simulink library "MIL_Test"  (Simulink 6.6)
undefined symbols (not defined in the file or in its folder): getdatatypespecs, slcm, StepSize
libraries: simulink x71, MIL_Test x6
(part 5 of 8)

== system MIL_Test/Validation Function/Feature extraction/Step response characteristics/Step response characteristics extraction/Extract maximum overshoot/Step response moving average and initial conditions before step ==
  Reset : Inport
  Step response : Inport  Port=2
  Add2 : Sum  Inputs=+-  OutScaling=2^-10
  Constant : Constant  Value=0
  Flip if new step : Subsystem  TreatAsAtomicUnit=on
  Memory : Memory
  Switch : Switch  Criteria=u2 ~= 0
  Switch1 : Switch  Criteria=u2 ~= 0
  Switch2 : Switch  Criteria=u2 ~= 0
  Weighted Moving Average : S-Function  FunctionName=sfix_fir  Parameters=(getdatatypespecs(OutDataType,OutScaling,DblOver,0)),[DoSatur RndMeth-1],DblOver,dolog,mgainval,(getdatatypespecs(GainDataType,GainScaling,DblOver,RadixGroup)),samptime,vinit,OutputDataTypeScalingMode,GainDataTypeScalingMode  mask(Weighted Moving Average){mgainval=ones(1,10), vinit=0.0, samptime=-1, GainDataTypeScalingMode=Inherit via internal rule, GainDataType=sfix( 16 ), MatRadixGroup=Best Precision: Matrix-wise, GainScaling=2^-10, OutputDataTypeScalingMode=Inherit via internal rule, OutDataType=sfix(16), OutScaling=2^-10, LockScale=off, RndMeth=Floor, DoSatur=off}
      mask prompts: mgainval "Weights:"; vinit "Initial condition:"; samptime "Sample time:"; GainDataTypeScalingMode "Gain data type and scaling:"; GainDataType "Parameter data type:     ex. sfix(16),  uint(8), float('single')"; MatRadixGroup "Parameter scaling mode:"; GainScaling "Parameter scaling:    Slope    ex.  2^-9"; OutputDataTypeScalingMode "Output data type and scaling:"; OutDataType "Output data type:     ex.  sfix(16),  uint(8),  float('single')"; OutScaling "Output scaling:    Slope or [Slope Bias]    ex.  2^-9"; LockScale "Lock output scaling so autoscaling tool can't change it"; RndMeth "Round toward:"; DoSatur "Saturate to max or min when overflows occur"
      mask help: Output the weighted moving average of the input.
      mask init: same as MIL_Test/Validation Function/Feature extraction/Step response characteristics/Step response characteristics extraction/Extract steady state error/Weighted Moving Average
      mask StyleString: edit,edit,edit,popup(Specify via dialog|Inherit via internal rule),edit,popup(Use Specified Scaling|Best Precision: Element-wise|Best Precision: Row-wise|Best Precision: Column-wise|Best Precision: Matrix-wise),edit,popup(Specify via dialog|Inherit via internal rule|Inherit via back propagation),edit,edit,checkbox,popup(Zero|Nearest|Ceiling|Floor),checkbox
      mask CallbackString: |||fixptdialog(gcbh)|fixptdialog(gcbh)|fixptdialog(gcbh)||fixptdialog(gcbh)|fixptdialog(gcbh)||||
      mask TabNameString: Main,Main,Main,Parameter data types,Parameter data types,Parameter data types,Parameter data types,Signal data types,Signal data types,Signal data types,Signal data types,Signal data types,Signal data types
      mask Display:
      | fprintf(fixpt_fir_mask_data(mgainval,'dispstr'))
      | plot(fixpt_fir_mask_data(mgainval,1),fixpt_fir_mask_data(mgainval,0))
  Weighted Moving Average1 : S-Function  FunctionName=sfix_fir  Parameters=(getdatatypespecs(OutDataType,OutScaling,DblOver,0)),[DoSatur RndMeth-1],DblOver,dolog,mgainval,(getdatatypespecs(GainDataType,GainScaling,DblOver,RadixGroup)),samptime,vinit,OutputDataTypeScalingMode,GainDataTypeScalingMode  mask(Weighted Moving Average){mgainval=ones(1,10), vinit=0.0, samptime=-1, GainDataTypeScalingMode=Inherit via internal rule, GainDataType=sfix( 16 ), MatRadixGroup=Best Precision: Matrix-wise, GainScaling=2^-10, OutputDataTypeScalingMode=Inherit via internal rule, OutDataType=sfix(16), OutScaling=2^-10, LockScale=off, RndMeth=Floor, DoSatur=off}
      mask prompts: mgainval "Weights:"; vinit "Initial condition:"; samptime "Sample time:"; GainDataTypeScalingMode "Gain data type and scaling:"; GainDataType "Parameter data type:     ex. sfix(16),  uint(8), float('single')"; MatRadixGroup "Parameter scaling mode:"; GainScaling "Parameter scaling:    Slope    ex.  2^-9"; OutputDataTypeScalingMode "Output data type and scaling:"; OutDataType "Output data type:     ex.  sfix(16),  uint(8),  float('single')"; OutScaling "Output scaling:    Slope or [Slope Bias]    ex.  2^-9"; LockScale "Lock output scaling so autoscaling tool can't change it"; RndMeth "Round toward:"; DoSatur "Saturate to max or min when overflows occur"
      mask help: Output the weighted moving average of the input.
      mask init: same as MIL_Test/Validation Function/Feature extraction/Step response characteristics/Step response characteristics extraction/Extract steady state error/Weighted Moving Average
      mask StyleString: edit,edit,edit,popup(Specify via dialog|Inherit via internal rule),edit,popup(Use Specified Scaling|Best Precision: Element-wise|Best Precision: Row-wise|Best Precision: Column-wise|Best Precision: Matrix-wise),edit,popup(Specify via dialog|Inherit via internal rule|Inherit via back propagation),edit,edit,checkbox,popup(Zero|Nearest|Ceiling|Floor),checkbox
      mask CallbackString: |||fixptdialog(gcbh)|fixptdialog(gcbh)|fixptdialog(gcbh)||fixptdialog(gcbh)|fixptdialog(gcbh)||||
      mask TabNameString: Main,Main,Main,Parameter data types,Parameter data types,Parameter data types,Parameter data types,Signal data types,Signal data types,Signal data types,Signal data types,Signal data types,Signal data types
      mask Display:
      | fprintf(fixpt_fir_mask_data(mgainval,'dispstr'))
      | plot(fixpt_fir_mask_data(mgainval,1),fixpt_fir_mask_data(mgainval,0))
  d(Step Response) average : Outport
  wires:
  Switch/1 -> d(Step Response) average/1
  Add2/1 -> Switch1/1, Switch2/3
  Constant/1 -> Switch2/1, Switch1/3
  Flip if new step/1(0/1) -> Switch2/2, Switch/2, Switch1/2
  Weighted Moving Average1/1 -> Switch/3
  Weighted Moving Average/1 -> Switch/1
  Switch2/1 -> Weighted Moving Average1/1
  Switch1/1 -> Weighted Moving Average/1
  Reset/1 -> Flip if new step/Enable
  Memory/1 -> Add2/2
  Step response/1 -> Add2/1, Memory/1

== system MIL_Test/Validation Function/Feature extraction/Step response characteristics/Step response characteristics extraction/Extract maximum overshoot/Trigger hold value ==
  d(Step Response) average : Inport
  Step sign : Inport  Port=2
  Add : Sum  OutScaling=2^-10
  Logical Operator1 : Logic  Operator=NOT  AllPortsSameDT=off  OutDataTypeMode=Boolean
  Negative step : Subsystem  mask(Compare To Zero){relop=>, LogicOutDataTypeMode=uint8, ZeroCross=off}
      mask prompts: relop "Operator:"; LogicOutDataTypeMode "Output data type mode:"; ZeroCross "Enable zero crossing detection"
      mask help: Determine how a signal compares to zero.
      mask init:
      | blkName = gcb;
      | 
      | if strcmp(get_param(gcbh,'LogicOutDataTypeMode'),'boolean')
      | 	setValue = 'Boolean';
      | else
      |     setValue = 'Specify via dialog';
      | end
      | 
      | set_param([blkName,'/Compare'],'relop',relop, ...
      | 	'LogicOutDataTypeMode', setValue, 'ZeroCross', ZeroCross);
      mask StyleString: popup(==|~=|<|<=|>=|>),popup(uint8|boolean),checkbox
      mask Display: disp([relop,' 0'])
  Positive step : Subsystem  mask(Compare To Zero){relop=<, LogicOutDataTypeMode=uint8, ZeroCross=off}
      mask prompts: relop "Operator:"; LogicOutDataTypeMode "Output data type mode:"; ZeroCross "Enable zero crossing detection"
      mask help: Determine how a signal compares to zero.
      mask init: same as MIL_Test/Validation Function/Feature extraction/Step response characteristics/Step response characteristics extraction/Extract maximum overshoot/Trigger hold value/Negative step
      mask StyleString: popup(==|~=|<|<=|>=|>),popup(uint8|boolean),checkbox
      mask Display: disp([relop,' 0'])
  Product : Product  RndMeth=Zero
  Product1 : Product  RndMeth=Zero
  Overshoot Trigger : Outport
  wires:
  Add/1 -> Overshoot Trigger/1
  Logical Operator1/1 -> Product/2
  Product1/1 -> Add/2
  Product/1 -> Add/1
  Step sign/1 -> Product1/1, Logical Operator1/1
  Positive step/1(y) -> Product1/2
  Negative step/1(y) -> Product/1
  d(Step Response) average/1 -> Positive step/1(u), Negative step/1(u)

== system MIL_Test/Validation Function/Feature extraction/Step response characteristics/Step response characteristics extraction/Extract rise time/Time difference ==
  Reset counter : Inport
  Clock : Inport  Port=2
  Trigger : TriggerPort  TriggerType=either
  Abs : Abs
  Execution counter : Subsystem  TreatAsAtomicUnit=on
  Memory : Memory  InheritSampleTime=on
  Memory1 : Memory  InheritSampleTime=on
  Number of executions : Constant  Value=3
  Relational Operator : RelationalOperator  Operator=<=  LogicOutDataTypeMode=Boolean
  Subtract : Sum  Inputs=+-  OutScaling=2^-10
  Switch : Switch  Criteria=u2 ~= 0
  Time difference : Outport
  wires:
  Execution counter/1(Counter) -> Relational Operator/1
  Reset counter/1 -> Execution counter/1(Reset)
  Number of executions/1 -> Relational Operator/2
  Abs/1 -> Time difference/1
  Subtract/1 -> Abs/1
  Relational Operator/1 -> Switch/2
  Memory1/1 -> Switch/3
  Memory/1 -> Memory1/1, Subtract/2
  Switch/1 -> Memory/1, Subtract/1
  Clock/1 -> Switch/1

== system MIL_Test/Validation Function/Feature extraction/Step response characteristics/Step response characteristics extraction/Extract settling time/Time stamp ==
  Clock : Inport
  Trigger : TriggerPort
  Time : Outport
  wires:
  Clock/1 -> Time/1

== system MIL_Test/Validation Function/Feature extraction/Step response characteristics/Step response reset/Active if signals constant for some specified time/Time since signal constant ==
  Signal : Inport
  Clock : Clock
      settings: Decimation=10
  Detect constant : Subsystem  TreatAsAtomicUnit=on  mask(Feature extraction block){RT=0.0001}
      mask prompts: RT "Relative tolerance in %"
      mask help: Detect if the signal value is constant (using the last two signal values) allowing for a user-defined relative deviation
      mask CallbackString:
      | if or( (str2double(get_param(gcb,'RT')) < 0), (str2double(get_param(gcb,'RT')) > 100))
      |     error(['Relative tolerance value (' get_param(gcb,'RT') ') out of range. Please give a value between 0 and 100.']);
      | else
      |     set_param([gcb '/Relative tolerance/Relative Tolerance'],'Value',get_param(gcb,'RT'));
      | end
  Logical Operator : Logic  Operator=NAND  AllPortsSameDT=off  OutDataTypeMode=Boolean
  Logical Operator1 : Logic  Operator=NOT  AllPortsSameDT=off  OutDataTypeMode=Boolean
  Memory : Memory  Orientation=left
  Memory1 : Memory
  Subtract : Sum  Inputs=-+  OutScaling=2^-10
  Switch : Switch  Criteria=u2 > Threshold
  Trigger : Outport
  Feature : Outport  Port=2
  wires:
  Logical Operator/1 -> Switch/2
  Logical Operator1/1 -> Logical Operator/2
  Memory1/1 -> Logical Operator1/1
  Memory/1 -> Switch/1
  Switch/1 -> Memory/1, Subtract/1
  Clock/1 -> Switch/3, Subtract/2
  Subtract/1 -> Feature/1
  Detect constant/1(Constant) -> Memory1/1, Logical Operator/1, Trigger/1
  Signal/1 -> Detect constant/1(Signal)

== system MIL_Test/Validation Function/Feature extraction/Step response characteristics/Step response reset/Active if signals constant for some specified time/Time since signal constant1 ==
  Signal : Inport
  Clock : Clock
      settings: Decimation=10
  Detect constant : Subsystem  TreatAsAtomicUnit=on  mask(Feature extraction block){RT=0.0001}
      mask prompts: RT "Relative tolerance in %"
      mask help: Detect if the signal value is constant (using the last two signal values) allowing for a user-defined relative deviation
      mask CallbackString:
      | if or( (str2double(get_param(gcb,'RT')) < 0), (str2double(get_param(gcb,'RT')) > 100))
      |     error(['Relative tolerance value (' get_param(gcb,'RT') ') out of range. Please give a value between 0 and 100.']);
      | else
      |     set_param([gcb '/Relative tolerance/Relative Tolerance'],'Value',get_param(gcb,'RT'));
      | end
  Logical Operator : Logic  Operator=NAND  AllPortsSameDT=off  OutDataTypeMode=Boolean
  Logical Operator1 : Logic  Operator=NOT  AllPortsSameDT=off  OutDataTypeMode=Boolean
  Memory : Memory  Orientation=left
  Memory1 : Memory
  Subtract : Sum  Inputs=-+  OutScaling=2^-10
  Switch : Switch  Criteria=u2 > Threshold
  Trigger : Outport
  Feature : Outport  Port=2
  wires:
  Signal/1 -> Detect constant/1(Signal)
  Detect constant/1(Constant) -> Trigger/1, Logical Operator/1, Memory1/1
  Subtract/1 -> Feature/1
  Clock/1 -> Subtract/2, Switch/3
  Switch/1 -> Subtract/1, Memory/1
  Memory/1 -> Switch/1
  Memory1/1 -> Logical Operator1/1
  Logical Operator1/1 -> Logical Operator/2
  Logical Operator/1 -> Switch/2

== system MIL_Test/Validation Function/Feature extraction/Step response characteristics/Step response trigger/Active if signals constant for some specified time/Time since signal constant ==
  Signal : Inport
  Clock : Clock
      settings: Decimation=10
  Detect constant : Subsystem  TreatAsAtomicUnit=on  mask(Feature extraction block){RT=0.5}
      mask prompts: RT "Relative tolerance in %"
      mask help: Detect if the signal value is constant (using the last two signal values) allowing for a user-defined relative deviation
      mask CallbackString:
      | if or( (str2double(get_param(gcb,'RT')) < 0), (str2double(get_param(gcb,'RT')) > 100))
      |     error(['Relative tolerance value (' get_param(gcb,'RT') ') out of range. Please give a value between 0 and 100.']);
      | else
      |     set_param([gcb '/Relative tolerance/Relative Tolerance'],'Value',get_param(gcb,'RT'));
      | end
  Logical Operator : Logic  Operator=NAND  AllPortsSameDT=off  OutDataTypeMode=Boolean
  Logical Operator1 : Logic  Operator=NOT  AllPortsSameDT=off  OutDataTypeMode=Boolean
  Memory : Memory  Orientation=left
  Memory1 : Memory
  Subtract : Sum  Inputs=-+  OutScaling=2^-10
  Switch : Switch  Criteria=u2 > Threshold
  Trigger : Outport
  Feature : Outport  Port=2
  wires:
  Logical Operator/1 -> Switch/2
  Logical Operator1/1 -> Logical Operator/2
  Memory1/1 -> Logical Operator1/1
  Memory/1 -> Switch/1
  Switch/1 -> Memory/1, Subtract/1
  Clock/1 -> Switch/3, Subtract/2
  Subtract/1 -> Feature/1
  Detect constant/1(Constant) -> Memory1/1, Logical Operator/1, Trigger/1
  Signal/1 -> Detect constant/1(Signal)

== system MIL_Test/Validation Function/Feature extraction/Step response characteristics/Step response trigger/Active if signals constant for some specified time/Time since signal constant1 ==
  Signal : Inport
  Clock : Clock
      settings: Decimation=10
  Detect constant : Subsystem  TreatAsAtomicUnit=on  mask(Feature extraction block){RT=0.5}
      mask prompts: RT "Relative tolerance in %"
      mask help: Detect if the signal value is constant (using the last two signal values) allowing for a user-defined relative deviation
      mask CallbackString:
      | if or( (str2double(get_param(gcb,'RT')) < 0), (str2double(get_param(gcb,'RT')) > 100))
      |     error(['Relative tolerance value (' get_param(gcb,'RT') ') out of range. Please give a value between 0 and 100.']);
      | else
      |     set_param([gcb '/Relative tolerance/Relative Tolerance'],'Value',get_param(gcb,'RT'));
      | end
  Logical Operator : Logic  Operator=NAND  AllPortsSameDT=off  OutDataTypeMode=Boolean
  Logical Operator1 : Logic  Operator=NOT  AllPortsSameDT=off  OutDataTypeMode=Boolean
  Memory : Memory  Orientation=left
  Memory1 : Memory
  Subtract : Sum  Inputs=-+  OutScaling=2^-10
  Switch : Switch  Criteria=u2 > Threshold
  Trigger : Outport
  Feature : Outport  Port=2
  wires:
  Signal/1 -> Detect constant/1(Signal)
  Detect constant/1(Constant) -> Trigger/1, Logical Operator/1, Memory1/1
  Subtract/1 -> Feature/1
  Clock/1 -> Subtract/2, Switch/3
  Switch/1 -> Subtract/1, Memory/1
  Memory/1 -> Switch/1
  Memory1/1 -> Logical Operator1/1
  Logical Operator1/1 -> Logical Operator/2
  Logical Operator/1 -> Switch/2

== system MIL_Test/Validation Function/TODO/<system name>/<Requirement name>/<Assertions name>/Feature extraction ==
  Sig : Inport
  R : Outport
  T : Outport  Port=2
  A : Outport  Port=3
  wires:
  Sig/1 -> A/1, T/1, R/1

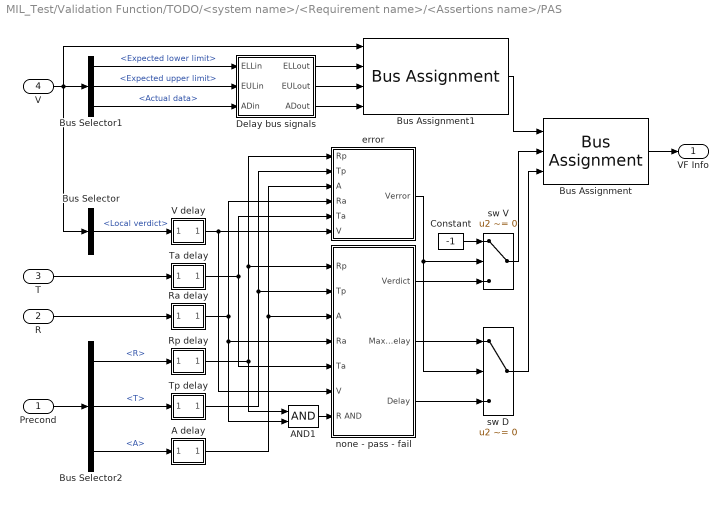
== system MIL_Test/Validation Function/TODO/<system name>/<Requirement name>/<Assertions name>/PAS ==
  Precond : Inport
  R : Inport  Port=2
  T : Inport  Port=3
  V : Inport  Port=4
  A delay : Subsystem  TreatAsAtomicUnit=on  mask{Delay=0}
      mask prompts: Delay "Delay (in simulation steps) for the input signal:"
      mask init:
      | %set_param([gcb '/Discrete Transfer Fcn'],'Denominator',['[' num2str([1 zeros(1,str2double(get_param(gcb,'Delay')))]) ']']);
      mask CallbackString:
      | Delay = str2double(get_param(gcb,'Delay'));
      | if Delay < 0
      |     set_param(gcb,'Delay','0');
      |     error('Only non-negative delays are possible (causality).');
      |     set_param([gcb '/Delay'],'Value','0');
      | elseif Delay == 0
      |     set_param([gcb '/Delay'],'Value','0');
      | else
      |     set_param([gcb '/Integer Delay'],'NumDelays',num2str(Delay));
      |     set_param([gcb '/Delay'],'Value',num2str(Delay));
      | end
      mask Display: text(0.5,0.5,['z^{ ' num2str((-1)*str2double(get_param(gcb,'Delay'))) '}'],'texmode','on');
  AND1 : Logic  AllPortsSameDT=off  OutDataTypeMode=Boolean
  Bus Selector : BusSelector  OutputSignals=Local verdict
  Bus Selector1 : BusSelector  OutputSignals=Expected lower limit,Expected upper limit,Actual data
  Bus Selector2 : BusSelector  OutputSignals=R,T,A
  Bus Assignment : BusAssignment  AssignedSignals=Local verdict,Delay
  Bus Assignment1 : BusAssignment  AssignedSignals=Expected lower limit,Expected upper limit,Actual data
  Constant : Constant  Value=-1
  Delay bus signals : Subsystem
  Ra delay : Subsystem  TreatAsAtomicUnit=on  mask{Delay=0}
      mask prompts: Delay "Delay (in simulation steps) for the input signal:"
      mask init:
      | %set_param([gcb '/Discrete Transfer Fcn'],'Denominator',['[' num2str([1 zeros(1,str2double(get_param(gcb,'Delay')))]) ']']);
      mask CallbackString:
      | Delay = str2double(get_param(gcb,'Delay'));
      | if Delay < 0
      |     set_param(gcb,'Delay','0');
      |     error('Only non-negative delays are possible (causality).');
      |     set_param([gcb '/Delay'],'Value','0');
      | elseif Delay == 0
      |     set_param([gcb '/Delay'],'Value','0');
      | else
      |     set_param([gcb '/Integer Delay'],'NumDelays',num2str(Delay));
      |     set_param([gcb '/Delay'],'Value',num2str(Delay));
      | end
      mask Display: text(0.5,0.5,['z^{ ' num2str((-1)*str2double(get_param(gcb,'Delay'))) '}'],'texmode','on');
  Rp delay : Subsystem  TreatAsAtomicUnit=on  mask{Delay=0}
      mask prompts: Delay "Delay (in simulation steps) for the input signal:"
      mask init:
      | %set_param([gcb '/Discrete Transfer Fcn'],'Denominator',['[' num2str([1 zeros(1,str2double(get_param(gcb,'Delay')))]) ']']);
      mask CallbackString:
      | Delay = str2double(get_param(gcb,'Delay'));
      | if Delay < 0
      |     set_param(gcb,'Delay','0');
      |     error('Only non-negative delays are possible (causality).');
      |     set_param([gcb '/Delay'],'Value','0');
      | elseif Delay == 0
      |     set_param([gcb '/Delay'],'Value','0');
      | else
      |     set_param([gcb '/Integer Delay'],'NumDelays',num2str(Delay));
      |     set_param([gcb '/Delay'],'Value',num2str(Delay));
      | end
      mask Display: text(0.5,0.5,['z^{ ' num2str((-1)*str2double(get_param(gcb,'Delay'))) '}'],'texmode','on');
  Ta delay : Subsystem  TreatAsAtomicUnit=on  mask{Delay=0}
      mask prompts: Delay "Delay (in simulation steps) for the input signal:"
      mask init:
      | %set_param([gcb '/Discrete Transfer Fcn'],'Denominator',['[' num2str([1 zeros(1,str2double(get_param(gcb,'Delay')))]) ']']);
      mask CallbackString:
      | Delay = str2double(get_param(gcb,'Delay'));
      | if Delay < 0
      |     set_param(gcb,'Delay','0');
      |     error('Only non-negative delays are possible (causality).');
      |     set_param([gcb '/Delay'],'Value','0');
      | elseif Delay == 0
      |     set_param([gcb '/Delay'],'Value','0');
      | else
      |     set_param([gcb '/Integer Delay'],'NumDelays',num2str(Delay));
      |     set_param([gcb '/Delay'],'Value',num2str(Delay));
      | end
      mask Display: text(0.5,0.5,['z^{ ' num2str((-1)*str2double(get_param(gcb,'Delay'))) '}'],'texmode','on');
  Tp delay : Subsystem  TreatAsAtomicUnit=on  mask{Delay=0}
      mask prompts: Delay "Delay (in simulation steps) for the input signal:"
      mask init:
      | %set_param([gcb '/Discrete Transfer Fcn'],'Denominator',['[' num2str([1 zeros(1,str2double(get_param(gcb,'Delay')))]) ']']);
      mask CallbackString:
      | Delay = str2double(get_param(gcb,'Delay'));
      | if Delay < 0
      |     set_param(gcb,'Delay','0');
      |     error('Only non-negative delays are possible (causality).');
      |     set_param([gcb '/Delay'],'Value','0');
      | elseif Delay == 0
      |     set_param([gcb '/Delay'],'Value','0');
      | else
      |     set_param([gcb '/Integer Delay'],'NumDelays',num2str(Delay));
      |     set_param([gcb '/Delay'],'Value',num2str(Delay));
      | end
      mask Display: text(0.5,0.5,['z^{ ' num2str((-1)*str2double(get_param(gcb,'Delay'))) '}'],'texmode','on');
  V delay : Subsystem  TreatAsAtomicUnit=on  mask{Delay=0}
      mask prompts: Delay "Delay (in simulation steps) for the input signal:"
      mask init:
      | %set_param([gcb '/Discrete Transfer Fcn'],'Denominator',['[' num2str([1 zeros(1,str2double(get_param(gcb,'Delay')))]) ']']);
      mask CallbackString:
      | Delay = str2double(get_param(gcb,'Delay'));
      | if Delay < 0
      |     set_param(gcb,'Delay','0');
      |     error('Only non-negative delays are possible (causality).');
      |     set_param([gcb '/Delay'],'Value','0');
      | elseif Delay == 0
      |     set_param([gcb '/Delay'],'Value','0');
      | else
      |     set_param([gcb '/Integer Delay'],'NumDelays',num2str(Delay));
      |     set_param([gcb '/Delay'],'Value',num2str(Delay));
      | end
      mask Display: text(0.5,0.5,['z^{ ' num2str((-1)*str2double(get_param(gcb,'Delay'))) '}'],'texmode','on');
  error : Subsystem
  none - pass - fail : Subsystem
  sw D : Switch  Criteria=u2 ~= 0
  sw V : Switch  Criteria=u2 ~= 0
  VF Info : Outport
  wires:
  V/1 -> Bus Selector/1, Bus Selector1/1, Bus Assignment1/1
  error/1(Verror) -> sw V/2, sw D/2
  Constant/1 -> sw V/1
  none - pass - fail/1(Verdict) -> sw V/3
  none - pass - fail/2(MaxDelay) -> sw D/1
  none - pass - fail/3(Delay) -> sw D/3
  sw V/1 -> Bus Assignment/2
  sw D/1 -> Bus Assignment/3
  Bus Selector/1 -> V delay/1(In1)  "<Local verdict>"
  Bus Assignment/1 -> VF Info/1
  Bus Selector2/1 -> Rp delay/1(In1)  "<R>"
  Bus Selector2/2 -> Tp delay/1(In1)  "<T>"
  Bus Selector2/3 -> A delay/1(In1)  "<A>"
  Rp delay/1(Out1) -> error/1(Rp), none - pass - fail/1(Rp), AND1/1
  Tp delay/1(Out1) -> error/2(Tp), none - pass - fail/2(Tp)
  A delay/1(Out1) -> error/3(A), none - pass - fail/3(A)
  V delay/1(Out1) -> error/6(V), none - pass - fail/6(V)
  Ra delay/1(Out1) -> none - pass - fail/4(Ra), AND1/2, error/4(Ra)
  AND1/1 -> none - pass - fail/7(R AND)
  Precond/1 -> Bus Selector2/1
  R/1 -> Ra delay/1(In1)
  T/1 -> Ta delay/1(In1)
  Bus Selector1/1 -> Delay bus signals/1(ELLin)  "<Expected lower limit>"
  Bus Selector1/2 -> Delay bus signals/2(EULin)  "<Expected upper limit>"
  Bus Selector1/3 -> Delay bus signals/3(ADin)  "<Actual data>"
  Bus Assignment1/1 -> Bus Assignment/1
  Delay bus signals/1(ELLout) -> Bus Assignment1/2
  Delay bus signals/2(EULout) -> Bus Assignment1/3
  Delay bus signals/3(ADout) -> Bus Assignment1/4
  Ta delay/1(Out1) -> none - pass - fail/5(Ta), error/5(Ta)

== system MIL_Test/Validation Function/TODO/<system name>/<Requirement name>/<Assertions name>/Signal comparison ==
  Sig : Inport
  Ref : Inport  Port=2
  Relational Operator : RelationalOperator  Operator=<=  LogicOutDataTypeMode=Boolean
  V : Outport
  wires:
  Relational Operator/1 -> V/1
  Sig/1 -> Relational Operator/1
  Ref/1 -> Relational Operator/2

== system MIL_Test/Validation Function/TODO/<system name>/<Requirement name>/<Preconditions name>/Feature extraction ==
  Sig : Inport
  R : Outport
  T : Outport  Port=2
  A : Outport  Port=3
  wires:
  Sig/1 -> R/1, T/1, A/1

== system MIL_Test/Validation Function/TODO/<system name>/<Requirement name>/<Preconditions name>/PS ==
  R TID1 : Inport
  T TID1 : Inport  Port=2
  A TID1 : Inport  Port=3
  AND : Logic  Inputs=4  AllPortsSameDT=off  OutDataTypeMode=Boolean
  Bus Creator : BusCreator  Inputs=3
  Data Type Conversion : DataTypeConversion
  Data Type Conversion1 : DataTypeConversion
  Data Type Conversion2 : DataTypeConversion
  Max Delay A : Subsystem  TreatAsAtomicUnit=on  mask{Delay=0}
      mask prompts: Delay "Delay (in simulation steps) for the input signal:"
      mask init:
      | %set_param([gcb '/Discrete Transfer Fcn'],'Denominator',['[' num2str([1 zeros(1,str2double(get_param(gcb,'Delay')))]) ']']);
      mask CallbackString:
      | Delay = str2double(get_param(gcb,'Delay'));
      | if Delay < 0
      |     set_param(gcb,'Delay','0');
      |     error('Only non-negative delays are possible (causality).');
      |     set_param([gcb '/Delay'],'Value','0');
      | elseif Delay == 0
      |     set_param([gcb '/Delay'],'Value','0');
      | else
      |     set_param([gcb '/Integer Delay'],'NumDelays',num2str(Delay));
      |     set_param([gcb '/Delay'],'Value',num2str(Delay));
      | end
      mask Display: text(0.5,0.5,['z^{ ' num2str((-1)*str2double(get_param(gcb,'Delay'))) '}'],'texmode','on');
  Max Delay R : Subsystem  TreatAsAtomicUnit=on  mask{Delay=0}
      mask prompts: Delay "Delay (in simulation steps) for the input signal:"
      mask init:
      | %set_param([gcb '/Discrete Transfer Fcn'],'Denominator',['[' num2str([1 zeros(1,str2double(get_param(gcb,'Delay')))]) ']']);
      mask CallbackString:
      | Delay = str2double(get_param(gcb,'Delay'));
      | if Delay < 0
      |     set_param(gcb,'Delay','0');
      |     error('Only non-negative delays are possible (causality).');
      |     set_param([gcb '/Delay'],'Value','0');
      | elseif Delay == 0
      |     set_param([gcb '/Delay'],'Value','0');
      | else
      |     set_param([gcb '/Integer Delay'],'NumDelays',num2str(Delay));
      |     set_param([gcb '/Delay'],'Value',num2str(Delay));
      | end
      mask Display: text(0.5,0.5,['z^{ ' num2str((-1)*str2double(get_param(gcb,'Delay'))) '}'],'texmode','on');
  Max Delay T : Subsystem  TreatAsAtomicUnit=on  mask{Delay=0}
      mask prompts: Delay "Delay (in simulation steps) for the input signal:"
      mask init:
      | %set_param([gcb '/Discrete Transfer Fcn'],'Denominator',['[' num2str([1 zeros(1,str2double(get_param(gcb,'Delay')))]) ']']);
      mask CallbackString:
      | Delay = str2double(get_param(gcb,'Delay'));
      | if Delay < 0
      |     set_param(gcb,'Delay','0');
      |     error('Only non-negative delays are possible (causality).');
      |     set_param([gcb '/Delay'],'Value','0');
      | elseif Delay == 0
      |     set_param([gcb '/Delay'],'Value','0');
      | else
      |     set_param([gcb '/Integer Delay'],'NumDelays',num2str(Delay));
      |     set_param([gcb '/Delay'],'Value',num2str(Delay));
      | end
      mask Display: text(0.5,0.5,['z^{ ' num2str((-1)*str2double(get_param(gcb,'Delay'))) '}'],'texmode','on');
  OR - AND : Subsystem
  TDD : Subsystem
  TI : Subsystem
  TID : Subsystem
  Precond : Outport
  wires:
  Data Type Conversion2/1 -> Bus Creator/3  "R"
  TI/1(A) -> AND/2
  OR - AND/1(OR) -> TID/3(R OR)
  OR - AND/2(AND) -> Max Delay R/1(In1), TID/4(R AND)
  AND/1 -> Data Type Conversion2/1
  Max Delay A/1(Out1) -> Data Type Conversion/1
  Max Delay R/1(Out1) -> AND/1
  Max Delay T/1(Out1) -> Data Type Conversion1/1
  TDD/1(A) -> AND/3
  Data Type Conversion1/1 -> Bus Creator/2  "T"
  Data Type Conversion/1 -> Bus Creator/1  "A"
  Bus Creator/1 -> Precond/1
  TID/1(A) -> Max Delay A/1(In1)
  TID/2(T) -> Max Delay T/1(In1)
  TDD/2(T) -> AND/4
  R TID1/1 -> OR - AND/1(R1)
  T TID1/1 -> TID/1(T1)
  A TID1/1 -> TID/2(A1)

== system MIL_Test/Validation Function/TODO/<system name>/<Requirement name>/<Preconditions name>/Signal comparison ==
  Sig : Inport
  Ref : Inport  Port=2
  Relational Operator : RelationalOperator  Operator=<=  LogicOutDataTypeMode=Boolean
  A : Outport
  wires:
  Ref/1 -> Relational Operator/2
  Sig/1 -> Relational Operator/1
  Relational Operator/1 -> A/1

== system MIL_Test/Validation Function/Test Evaluation Architecture/<system name>/<Requirement name>/<Assertions name>/Feature extraction ==
  Sig : Inport
  R : Outport
  T : Outport  Port=2
  A : Outport  Port=3
  wires:
  Sig/1 -> R/1, T/1, A/1

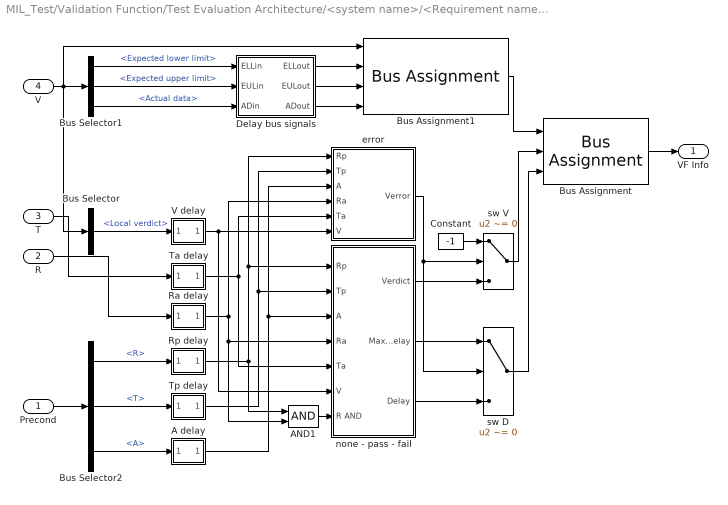
== system MIL_Test/Validation Function/Test Evaluation Architecture/<system name>/<Requirement name>/<Assertions name>/PAS ==
  Precond : Inport
  R : Inport  Port=2
  T : Inport  Port=3
  V : Inport  Port=4
  A delay : Subsystem  TreatAsAtomicUnit=on  mask{Delay=600}
      mask prompts: Delay "Delay (in simulation steps) for the input signal:"
      mask init:
      | %set_param([gcb '/Discrete Transfer Fcn'],'Denominator',['[' num2str([1 zeros(1,str2double(get_param(gcb,'Delay')))]) ']']);
      mask CallbackString:
      | Delay = str2double(get_param(gcb,'Delay'));
      | if Delay < 0
      |     set_param(gcb,'Delay','0');
      |     error('Only non-negative delays are possible (causality).');
      |     set_param([gcb '/Delay'],'Value','0');
      | elseif Delay == 0
      |     set_param([gcb '/Delay'],'Value','0');
      | else
      |     set_param([gcb '/Integer Delay'],'NumDelays',num2str(Delay));
      |     set_param([gcb '/Delay'],'Value',num2str(Delay));
      | end
      mask Display: text(0.5,0.5,['z^{ ' num2str((-1)*str2double(get_param(gcb,'Delay'))) '}'],'texmode','on');
  AND1 : Logic  AllPortsSameDT=off  OutDataTypeMode=Boolean
  Bus Selector : BusSelector  OutputSignals=Local verdict
  Bus Selector1 : BusSelector  OutputSignals=Expected lower limit,Expected upper limit,Actual data
  Bus Selector2 : BusSelector  OutputSignals=R,T,A
  Bus Assignment : BusAssignment  AssignedSignals=Local verdict,Delay
  Bus Assignment1 : BusAssignment  AssignedSignals=Expected lower limit,Expected upper limit,Actual data
  Constant : Constant  Value=-1
  Delay bus signals : Subsystem
  Ra delay : Subsystem  TreatAsAtomicUnit=on  mask{Delay=0}
      mask prompts: Delay "Delay (in simulation steps) for the input signal:"
      mask init:
      | %set_param([gcb '/Discrete Transfer Fcn'],'Denominator',['[' num2str([1 zeros(1,str2double(get_param(gcb,'Delay')))]) ']']);
      mask CallbackString:
      | Delay = str2double(get_param(gcb,'Delay'));
      | if Delay < 0
      |     set_param(gcb,'Delay','0');
      |     error('Only non-negative delays are possible (causality).');
      |     set_param([gcb '/Delay'],'Value','0');
      | elseif Delay == 0
      |     set_param([gcb '/Delay'],'Value','0');
      | else
      |     set_param([gcb '/Integer Delay'],'NumDelays',num2str(Delay));
      |     set_param([gcb '/Delay'],'Value',num2str(Delay));
      | end
      mask Display: text(0.5,0.5,['z^{ ' num2str((-1)*str2double(get_param(gcb,'Delay'))) '}'],'texmode','on');
  Rp delay : Subsystem  TreatAsAtomicUnit=on  mask{Delay=600}
      mask prompts: Delay "Delay (in simulation steps) for the input signal:"
      mask init:
      | %set_param([gcb '/Discrete Transfer Fcn'],'Denominator',['[' num2str([1 zeros(1,str2double(get_param(gcb,'Delay')))]) ']']);
      mask CallbackString:
      | Delay = str2double(get_param(gcb,'Delay'));
      | if Delay < 0
      |     set_param(gcb,'Delay','0');
      |     error('Only non-negative delays are possible (causality).');
      |     set_param([gcb '/Delay'],'Value','0');
      | elseif Delay == 0
      |     set_param([gcb '/Delay'],'Value','0');
      | else
      |     set_param([gcb '/Integer Delay'],'NumDelays',num2str(Delay));
      |     set_param([gcb '/Delay'],'Value',num2str(Delay));
      | end
      mask Display: text(0.5,0.5,['z^{ ' num2str((-1)*str2double(get_param(gcb,'Delay'))) '}'],'texmode','on');
  Ta delay : Subsystem  TreatAsAtomicUnit=on  mask{Delay=0}
      mask prompts: Delay "Delay (in simulation steps) for the input signal:"
      mask init:
      | %set_param([gcb '/Discrete Transfer Fcn'],'Denominator',['[' num2str([1 zeros(1,str2double(get_param(gcb,'Delay')))]) ']']);
      mask CallbackString:
      | Delay = str2double(get_param(gcb,'Delay'));
      | if Delay < 0
      |     set_param(gcb,'Delay','0');
      |     error('Only non-negative delays are possible (causality).');
      |     set_param([gcb '/Delay'],'Value','0');
      | elseif Delay == 0
      |     set_param([gcb '/Delay'],'Value','0');
      | else
      |     set_param([gcb '/Integer Delay'],'NumDelays',num2str(Delay));
      |     set_param([gcb '/Delay'],'Value',num2str(Delay));
      | end
      mask Display: text(0.5,0.5,['z^{ ' num2str((-1)*str2double(get_param(gcb,'Delay'))) '}'],'texmode','on');
  Tp delay : Subsystem  TreatAsAtomicUnit=on  mask{Delay=600}
      mask prompts: Delay "Delay (in simulation steps) for the input signal:"
      mask init:
      | %set_param([gcb '/Discrete Transfer Fcn'],'Denominator',['[' num2str([1 zeros(1,str2double(get_param(gcb,'Delay')))]) ']']);
      mask CallbackString:
      | Delay = str2double(get_param(gcb,'Delay'));
      | if Delay < 0
      |     set_param(gcb,'Delay','0');
      |     error('Only non-negative delays are possible (causality).');
      |     set_param([gcb '/Delay'],'Value','0');
      | elseif Delay == 0
      |     set_param([gcb '/Delay'],'Value','0');
      | else
      |     set_param([gcb '/Integer Delay'],'NumDelays',num2str(Delay));
      |     set_param([gcb '/Delay'],'Value',num2str(Delay));
      | end
      mask Display: text(0.5,0.5,['z^{ ' num2str((-1)*str2double(get_param(gcb,'Delay'))) '}'],'texmode','on');
  V delay : Subsystem  TreatAsAtomicUnit=on  mask{Delay=0}
      mask prompts: Delay "Delay (in simulation steps) for the input signal:"
      mask init:
      | %set_param([gcb '/Discrete Transfer Fcn'],'Denominator',['[' num2str([1 zeros(1,str2double(get_param(gcb,'Delay')))]) ']']);
      mask CallbackString:
      | Delay = str2double(get_param(gcb,'Delay'));
      | if Delay < 0
      |     set_param(gcb,'Delay','0');
      |     error('Only non-negative delays are possible (causality).');
      |     set_param([gcb '/Delay'],'Value','0');
      | elseif Delay == 0
      |     set_param([gcb '/Delay'],'Value','0');
      | else
      |     set_param([gcb '/Integer Delay'],'NumDelays',num2str(Delay));
      |     set_param([gcb '/Delay'],'Value',num2str(Delay));
      | end
      mask Display: text(0.5,0.5,['z^{ ' num2str((-1)*str2double(get_param(gcb,'Delay'))) '}'],'texmode','on');
  error : Subsystem
  none - pass - fail : Subsystem
  sw D : Switch  Criteria=u2 ~= 0
  sw V : Switch  Criteria=u2 ~= 0
  VF Info : Outport
  wires:
  Ta delay/1(Out1) -> error/5(Ta), none - pass - fail/5(Ta)
  Delay bus signals/3(ADout) -> Bus Assignment1/4
  Delay bus signals/2(EULout) -> Bus Assignment1/3
  Delay bus signals/1(ELLout) -> Bus Assignment1/2
  Bus Assignment1/1 -> Bus Assignment/1
  Bus Selector1/3 -> Delay bus signals/3(ADin)  "<Actual data>"
  Bus Selector1/2 -> Delay bus signals/2(EULin)  "<Expected upper limit>"
  Bus Selector1/1 -> Delay bus signals/1(ELLin)  "<Expected lower limit>"
  Precond/1 -> Bus Selector2/1
  AND1/1 -> none - pass - fail/7(R AND)
  Ra delay/1(Out1) -> error/4(Ra), AND1/2, none - pass - fail/4(Ra)
  V delay/1(Out1) -> none - pass - fail/6(V), error/6(V)
  A delay/1(Out1) -> none - pass - fail/3(A), error/3(A)
  Tp delay/1(Out1) -> none - pass - fail/2(Tp), error/2(Tp)
  Rp delay/1(Out1) -> AND1/1, none - pass - fail/1(Rp), error/1(Rp)
  Bus Selector2/3 -> A delay/1(In1)  "<A>"
  Bus Selector2/2 -> Tp delay/1(In1)  "<T>"
  Bus Selector2/1 -> Rp delay/1(In1)  "<R>"
  Bus Assignment/1 -> VF Info/1
  Bus Selector/1 -> V delay/1(In1)  "<Local verdict>"
  sw D/1 -> Bus Assignment/3
  sw V/1 -> Bus Assignment/2
  none - pass - fail/3(Delay) -> sw D/3
  none - pass - fail/2(MaxDelay) -> sw D/1
  none - pass - fail/1(Verdict) -> sw V/3
  Constant/1 -> sw V/1
  error/1(Verror) -> sw D/2, sw V/2
  V/1 -> Bus Assignment1/1, Bus Selector1/1, Bus Selector/1
  R/1 -> Ra delay/1(In1)
  T/1 -> Ta delay/1(In1)

== system MIL_Test/Validation Function/Test Evaluation Architecture/<system name>/<Requirement name>/<Assertions name>/Signal comparison ==
  Sig : Inport
  Ref : Inport  Port=2
  Relational Operator : RelationalOperator  Operator=<=  LogicOutDataTypeMode=Boolean
  V : Outport
  wires:
  Ref/1 -> Relational Operator/2
  Sig/1 -> Relational Operator/1
  Relational Operator/1 -> V/1

== system MIL_Test/Validation Function/Test Evaluation Architecture/<system name>/<Requirement name>/<Preconditions name>/Feature extraction ==
  Sig : Inport
  R : Outport
  T : Outport  Port=2
  A : Outport  Port=3
  wires:
  Sig/1 -> A/1, T/1, R/1

== system MIL_Test/Validation Function/Test Evaluation Architecture/<system name>/<Requirement name>/<Preconditions name>/PS ==
  R TID1 : Inport
  T TID1 : Inport  Port=2
  A TID1 : Inport  Port=3
  AND : Logic  Inputs=4  AllPortsSameDT=off  OutDataTypeMode=Boolean
  Bus Creator : BusCreator  Inputs=3
  Data Type Conversion : DataTypeConversion
  Data Type Conversion1 : DataTypeConversion
  Data Type Conversion2 : DataTypeConversion
  Max Delay A : Subsystem  TreatAsAtomicUnit=on  mask{Delay=0}
      mask prompts: Delay "Delay (in simulation steps) for the input signal:"
      mask init:
      | %set_param([gcb '/Discrete Transfer Fcn'],'Denominator',['[' num2str([1 zeros(1,str2double(get_param(gcb,'Delay')))]) ']']);
      mask CallbackString:
      | Delay = str2double(get_param(gcb,'Delay'));
      | if Delay < 0
      |     set_param(gcb,'Delay','0');
      |     error('Only non-negative delays are possible (causality).');
      |     set_param([gcb '/Delay'],'Value','0');
      | elseif Delay == 0
      |     set_param([gcb '/Delay'],'Value','0');
      | else
      |     set_param([gcb '/Integer Delay'],'NumDelays',num2str(Delay));
      |     set_param([gcb '/Delay'],'Value',num2str(Delay));
      | end
      mask Display: text(0.5,0.5,['z^{ ' num2str((-1)*str2double(get_param(gcb,'Delay'))) '}'],'texmode','on');
  Max Delay R : Subsystem  TreatAsAtomicUnit=on  mask{Delay=0}
      mask prompts: Delay "Delay (in simulation steps) for the input signal:"
      mask init:
      | %set_param([gcb '/Discrete Transfer Fcn'],'Denominator',['[' num2str([1 zeros(1,str2double(get_param(gcb,'Delay')))]) ']']);
      mask CallbackString:
      | Delay = str2double(get_param(gcb,'Delay'));
      | if Delay < 0
      |     set_param(gcb,'Delay','0');
      |     error('Only non-negative delays are possible (causality).');
      |     set_param([gcb '/Delay'],'Value','0');
      | elseif Delay == 0
      |     set_param([gcb '/Delay'],'Value','0');
      | else
      |     set_param([gcb '/Integer Delay'],'NumDelays',num2str(Delay));
      |     set_param([gcb '/Delay'],'Value',num2str(Delay));
      | end
      mask Display: text(0.5,0.5,['z^{ ' num2str((-1)*str2double(get_param(gcb,'Delay'))) '}'],'texmode','on');
  Max Delay T : Subsystem  TreatAsAtomicUnit=on  mask{Delay=0}
      mask prompts: Delay "Delay (in simulation steps) for the input signal:"
      mask init:
      | %set_param([gcb '/Discrete Transfer Fcn'],'Denominator',['[' num2str([1 zeros(1,str2double(get_param(gcb,'Delay')))]) ']']);
      mask CallbackString:
      | Delay = str2double(get_param(gcb,'Delay'));
      | if Delay < 0
      |     set_param(gcb,'Delay','0');
      |     error('Only non-negative delays are possible (causality).');
      |     set_param([gcb '/Delay'],'Value','0');
      | elseif Delay == 0
      |     set_param([gcb '/Delay'],'Value','0');
      | else
      |     set_param([gcb '/Integer Delay'],'NumDelays',num2str(Delay));
      |     set_param([gcb '/Delay'],'Value',num2str(Delay));
      | end
      mask Display: text(0.5,0.5,['z^{ ' num2str((-1)*str2double(get_param(gcb,'Delay'))) '}'],'texmode','on');
  OR - AND : Subsystem
  TDD : Subsystem
  TI : Subsystem
  TID : Subsystem
  Precond : Outport
  wires:
  A TID1/1 -> TID/2(A1)
  T TID1/1 -> TID/1(T1)
  R TID1/1 -> OR - AND/1(R1)
  TDD/2(T) -> AND/4
  TID/2(T) -> Max Delay T/1(In1)
  TID/1(A) -> Max Delay A/1(In1)
  Bus Creator/1 -> Precond/1
  Data Type Conversion/1 -> Bus Creator/1  "A"
  Data Type Conversion1/1 -> Bus Creator/2  "T"
  TDD/1(A) -> AND/3
  Max Delay T/1(Out1) -> Data Type Conversion1/1
  Max Delay R/1(Out1) -> AND/1
  Max Delay A/1(Out1) -> Data Type Conversion/1
  AND/1 -> Data Type Conversion2/1
  OR - AND/2(AND) -> TID/4(R AND), Max Delay R/1(In1)
  OR - AND/1(OR) -> TID/3(R OR)
  TI/1(A) -> AND/2
  Data Type Conversion2/1 -> Bus Creator/3  "R"

== system MIL_Test/Validation Function/Test Evaluation Architecture/<system name>/<Requirement name>/<Preconditions name>/Signal comparison ==
  Sig : Inport
  Ref : Inport  Port=2
  Relational Operator : RelationalOperator  Operator=<=  LogicOutDataTypeMode=Boolean
  A : Outport
  wires:
  Relational Operator/1 -> A/1
  Sig/1 -> Relational Operator/1
  Ref/1 -> Relational Operator/2

== system MIL_Test/Test Control/Test Control Architecture/Connection Helpers/TestControl for  TestCases Sequencing NoMask/IF Signal@SimStopTime for TC = value1/if Signal@t for TC = pass/check in range ==
  @[time] : Inport
  Signal : Inport  Port=2
  Enable : EnablePort
  Logical Operator2 : Logic  AllPortsSameDT=off  OutDataTypeMode=Boolean
  Relational Operator : RelationalOperator  Operator===  LogicOutDataTypeMode=Boolean
  Value : Constant  Value=condition
  Control Seq : Outport  InitialOutput=[2]
  wires:
  Signal/1 -> Relational Operator/1
  Value/1 -> Relational Operator/2
  Relational Operator/1 -> Logical Operator2/1
  Logical Operator2/1 -> Control Seq/1
  @[time]/1 -> Logical Operator2/2

== system MIL_Test/Test Control/Test Control Architecture/Connection Helpers/TestControl for  TestCases Sequencing NoMask/IF signal @[timeUp, timeDown] for TC = value1/if Signal@ [TDown,TUp]  for TC = Value/check in range ==
  @[time] : Inport
  Signal : Inport  Port=2
  Enable : EnablePort
  Logical Operator2 : Logic  AllPortsSameDT=off  OutDataTypeMode=Boolean
  Relational Operator : RelationalOperator  Operator===  LogicOutDataTypeMode=Boolean
  Value : Constant  Value=condition
  Control Seq : Outport  InitialOutput=[2]
  wires:
  Signal/1 -> Relational Operator/1
  Value/1 -> Relational Operator/2
  Relational Operator/1 -> Logical Operator2/1
  Logical Operator2/1 -> Control Seq/1
  @[time]/1 -> Logical Operator2/2

== system MIL_Test/Test Control/Test Control Architecture/Connection Helpers/TestControl for  TestCases Sequencing NoMask/IF signal@time for TC = value1/if Signal@t for TC = pass/check in range ==
  @[time] : Inport
  Signal : Inport  Port=2
  Enable : EnablePort
  Logical Operator2 : Logic  AllPortsSameDT=off  OutDataTypeMode=Boolean
  Relational Operator : RelationalOperator  Operator===  LogicOutDataTypeMode=Boolean
  Value : Constant  Value=condition
  Control Seq : Outport  InitialOutput=[2]
  wires:
  Signal/1 -> Relational Operator/1
  Value/1 -> Relational Operator/2
  Relational Operator/1 -> Logical Operator2/1
  Logical Operator2/1 -> Control Seq/1
  @[time]/1 -> Logical Operator2/2

== system MIL_Test/Test Data/Test Data Architecture/<Test data generator>/<Requirement name>/<Preconditions name>/<Check>/Signal comparison ==
  Sig : Inport
  Ref : Inport  Port=2
  Relational Operator : RelationalOperator  Operator=<=  LogicOutDataTypeMode=Boolean
  A : Outport
  wires:
  Relational Operator/1 -> A/1
  Sig/1 -> Relational Operator/1
  Ref/1 -> Relational Operator/2

== system MIL_Test/Validation Function/Feature extraction/Complete step detection/Step detection/Active if signals constant for some specified time/Time since signal constant/Detect constant ==
  Signal : Inport
  Clock : Clock
      settings: Decimation=10
  Constant1 : Constant  Value=0  OutDataTypeMode=boolean
  Memory : Memory
  Relative tolerance : Subsystem
  Switch : Switch  Criteria=u2 > Threshold
  Constant : Outport
  wires:
  Switch/1 -> Constant/1
  Relative tolerance/1(sig == ref) -> Switch/1
  Clock/1 -> Switch/2
  Constant1/1 -> Switch/3
  Memory/1 -> Relative tolerance/2(ref)
  Signal/1 -> Relative tolerance/1(sig), Memory/1

== system MIL_Test/Validation Function/Feature extraction/Complete step detection/Step detection/Active if signals constant for some specified time/Time since signal constant1/Detect constant ==
  Signal : Inport
  Clock : Clock
      settings: Decimation=10
  Constant1 : Constant  Value=0  OutDataTypeMode=boolean
  Memory : Memory
  Relative tolerance : Subsystem
  Switch : Switch  Criteria=u2 > Threshold
  Constant : Outport
  wires:
  Signal/1 -> Relative tolerance/1(sig), Memory/1
  Memory/1 -> Relative tolerance/2(ref)
  Constant1/1 -> Switch/3
  Clock/1 -> Switch/2
  Relative tolerance/1(sig == ref) -> Switch/1
  Switch/1 -> Constant/1

== system MIL_Test/Validation Function/Feature extraction/Complete step detection/Step detection reset/Active if signals constant for some specified time/Time since signal constant/Detect constant ==
  Signal : Inport
  Clock : Clock
      settings: Decimation=10
  Constant1 : Constant  Value=0  OutDataTypeMode=boolean
  Memory : Memory
  Relative tolerance : Subsystem
  Switch : Switch  Criteria=u2 > Threshold
  Constant : Outport
  wires:
  Switch/1 -> Constant/1
  Relative tolerance/1(sig == ref) -> Switch/1
  Clock/1 -> Switch/2
  Constant1/1 -> Switch/3
  Memory/1 -> Relative tolerance/2(ref)
  Signal/1 -> Relative tolerance/1(sig), Memory/1

== system MIL_Test/Validation Function/Feature extraction/Complete step detection/Step detection reset/Active if signals constant for some specified time/Time since signal constant1/Detect constant ==
  Signal : Inport
  Clock : Clock
      settings: Decimation=10
  Constant1 : Constant  Value=0  OutDataTypeMode=boolean
  Memory : Memory
  Relative tolerance : Subsystem
  Switch : Switch  Criteria=u2 > Threshold
  Constant : Outport
  wires:
  Signal/1 -> Relative tolerance/1(sig), Memory/1
  Memory/1 -> Relative tolerance/2(ref)
  Constant1/1 -> Switch/3
  Clock/1 -> Switch/2
  Relative tolerance/1(sig == ref) -> Switch/1
  Switch/1 -> Constant/1

== system MIL_Test/Validation Function/Feature extraction/Step response characteristics/Step response characteristics extraction/Extract maximum overshoot/Active if signals constant for some specified time/Time since signal constant ==
  Signal : Inport
  Clock : Clock
      settings: Decimation=10
  Detect constant : Subsystem  TreatAsAtomicUnit=on  mask(Feature extraction block){RT=0.1}
      mask prompts: RT "Relative tolerance in %"
      mask help: Detect if the signal value is constant (using the last two signal values) allowing for a user-defined relative deviation
      mask CallbackString:
      | if or( (str2double(get_param(gcb,'RT')) < 0), (str2double(get_param(gcb,'RT')) > 100))
      |     error(['Relative tolerance value (' get_param(gcb,'RT') ') out of range. Please give a value between 0 and 100.']);
      | else
      |     set_param([gcb '/Relative tolerance/Relative Tolerance'],'Value',get_param(gcb,'RT'));
      | end
  Logical Operator : Logic  Operator=NAND  AllPortsSameDT=off  OutDataTypeMode=Boolean
  Logical Operator1 : Logic  Operator=NOT  AllPortsSameDT=off  OutDataTypeMode=Boolean
  Memory : Memory  Orientation=left
  Memory1 : Memory
  Subtract : Sum  Inputs=-+  OutScaling=2^-10
  Switch : Switch  Criteria=u2 > Threshold
  Trigger : Outport
  Feature : Outport  Port=2
  wires:
  Logical Operator/1 -> Switch/2
  Logical Operator1/1 -> Logical Operator/2
  Memory1/1 -> Logical Operator1/1
  Memory/1 -> Switch/1
  Switch/1 -> Memory/1, Subtract/1
  Clock/1 -> Switch/3, Subtract/2
  Subtract/1 -> Feature/1
  Detect constant/1(Constant) -> Memory1/1, Logical Operator/1, Trigger/1
  Signal/1 -> Detect constant/1(Signal)
